simulink model "sampleModel7293_pp_1_1"  (R2018a)
settings: Solver=VariableStepAuto  StartTime=0.0  StopTime=10.0  RelTol=1e-3
undefined symbols (not defined in the file): DiscIntNeverNeededParam
libraries: simulink x367
(part 6 of 12)

== system sampleModel7293_pp_1_1/cfblk167/cfblk17 ==
  cfblk1 : Inport
  Action Port : ActionPort  ActionType=then
  cfblk3 : DiscreteTransferFcn
  cfblk4 : DiscreteIntegrator  SampleTime=-1  OutDataTypeStr=double  ICPrevOutput=DiscIntNeverNeededParam  ICPrevScaledInput=DiscIntNeverNeededParam
  cfblk5 : Subsystem  TreatAsAtomicUnit=on
  cfblk6 : DiscreteZeroPole  Poles=[0 0.5]  Gain=1  SampleTime=-1
  cfblk7 : Subsystem  TreatAsAtomicUnit=on
  cyemi_{112..116} (5 alike) : DataTypeConversion  OutDataTypeStr=double
  emi_417 : Subsystem  TreatAsAtomicUnit=on
  emi_419 : If  IfExpression=Inf <= u1
  emi_420 : DataTypeConversion  OutDataTypeStr=double
  emi_533 : Subsystem  TreatAsAtomicUnit=on
  emi_535 : If  IfExpression=Inf <= u1
  emi_536 : DataTypeConversion  OutDataTypeStr=double
  cfblk2 : Outport
  wires:
  cyemi_112/1 -> cfblk3/1
  cfblk1/1 -> cyemi_112/1
  cyemi_113/1 -> cfblk4/1
  cfblk6/1 -> cyemi_113/1
  cfblk3/1 -> cyemi_114/1, emi_420/1, emi_536/1
  cyemi_115/1 -> cfblk6/1
  cfblk4/1 -> cyemi_116/1
  cyemi_114/1 -> cfblk5/1(emi_415)
  cfblk5/1(emi_416) -> cyemi_115/1
  emi_419/1 -> cfblk5/Action
  emi_419/2 -> emi_417/Action
  emi_420/1 -> emi_419/1
  cyemi_116/1 -> cfblk7/1(emi_531)
  cfblk7/1(emi_532) -> cfblk2/1
  emi_535/1 -> cfblk7/Action
  emi_535/2 -> emi_533/Action
  emi_536/1 -> emi_535/1

== system sampleModel7293_pp_1_1/cfblk167/cfblk18 ==
  cfblk1 : Inport
  cfblk10 : Inport  Port=2
  cfblk11 : Inport  Port=3
  Action Port : ActionPort  ActionType=else
  cfblk14 : Delay
  cfblk3 : simulink/Discrete/Transfer Fcn Lead or Lag  PoleZ=0.95  ZeroZ=0.75  ICPrevOutput=0.0  ICPrevInput=0.0  DoSatur=off
      settings: SourceProductName=Simulink  SourceProductBaseCode=SL
  cfblk4 : Subsystem  TreatAsAtomicUnit=on
  cfblk5 : simulink/Discrete/Tapped Delay  vinit=0.0  samptime=-1  NumDelays=1  DelayOrder=Oldest  includeCurrent=off
  cfblk6 : Subsystem  TreatAsAtomicUnit=on
  cfblk7 : Delay
  cfblk8 : Subsystem  TreatAsAtomicUnit=on
  cfblk9 : DiscreteFir
  cyemi_{120..127} (8 alike) : DataTypeConversion  OutDataTypeStr=double
  emi_1559 : Subsystem  TreatAsAtomicUnit=on
  emi_1561 : If  IfExpression=0 <= u1
  emi_1562 : DataTypeConversion  OutDataTypeStr=double
  emi_2121 : Subsystem  TreatAsAtomicUnit=on
  emi_2123 : If  IfExpression=0 <= u1
  emi_2124 : DataTypeConversion  OutDataTypeStr=double
  emi_38 : Subsystem  TreatAsAtomicUnit=on
  emi_40 : If  IfExpression=0 <= u1
  emi_41 : DataTypeConversion  OutDataTypeStr=double
  cfblk2 : Outport
  cfblk12 : Outport  Port=2
  cfblk13 : Outport  Port=3
  wires:
  cfblk1/1 -> cfblk12/1
  cfblk5/1 -> cfblk2/1, emi_41/1
  cyemi_120/1 -> cfblk14/1
  cfblk9/1 -> cyemi_120/1
  cyemi_121/1 -> cfblk3/1
  cfblk11/1 -> cyemi_121/1
  cyemi_123/1 -> cfblk5/1
  cfblk3/1 -> cyemi_124/1
  cyemi_125/1 -> cfblk7/1
  cfblk14/1 -> cyemi_125/1
  cfblk10/1 -> cyemi_126/1
  cyemi_127/1 -> cfblk9/1
  cfblk7/1 -> cyemi_127/1, emi_2124/1
  cyemi_126/1 -> cfblk8/1(emi_36)
  cfblk8/1(emi_37) -> cfblk13/1, emi_1562/1
  emi_40/1 -> cfblk8/Action
  emi_40/2 -> emi_38/Action
  emi_41/1 -> emi_40/1
  cyemi_122/1 -> cfblk4/1(emi_1557)
  cfblk4/1(emi_1558) -> cyemi_123/1
  emi_1561/1 -> cfblk4/Action
  emi_1561/2 -> emi_1559/Action
  emi_1562/1 -> emi_1561/1
  cyemi_124/1 -> cfblk6/1(emi_2119)
  cfblk6/1(emi_2120) -> cyemi_122/1
  emi_2123/1 -> cfblk6/Action
  emi_2123/2 -> emi_2121/Action
  emi_2124/1 -> emi_2123/1

== system sampleModel7293_pp_1_1/cfblk167/cfblk19 ==
  cfblk1 : Inport
  Action Port : ActionPort  ActionType=then
  cfblk10 : Delay
  cfblk3 : Delay  ShowEnablePort=on
      settings: InputPortMap=u0,e6
  cfblk4 : simulink/Discrete/Transfer Fcn Real Zero  ZeroZ=0.75  ICPrevInput=0.0  DoSatur=off
      settings: SourceProductName=Simulink  SourceProductBaseCode=SL
  cfblk5 : DiscreteZeroPole  Poles=[0 0.5]  Gain=1  SampleTime=-1
  cfblk6 : simulink/Continuous/PID Controller  Controller=PID  TimeDomain=Discrete-time  SampleTime=-1  IntegratorMethod=Forward Euler  FilterMethod=Forward Euler  Form=Parallel  UseFilter=on  ControllerParametersSource=internal  P=1  I=1  D=0  N=100  InitialConditionSource=internal  InitialConditionForIntegrator=0  InitialConditionForFilter=0  ExternalReset=none  LimitOutput=off  UpperSaturationLimit=inf  LowerSaturationLimit=-inf  LinearizeAsGain=off  AntiWindupMode=none  Kb=1  TrackingMode=off  Kt=1  PParamMin=[]  PParamMax=[]  IParamMin=[]  IParamMax=[]  DParamMin=[]  DParamMax=[]  NParamMin=[]  NParamMax=[]  KbParamMin=[]  KbParamMax=[]  KtParamMin=[]  KtParamMax=[]  POutMin=[]  POutMax=[]  IOutMin=[]  IOutMax=[]  DOutMin=[]  DOutMax=[]  NOutMin=[]  NOutMax=[]  KbOutMin=[]  KbOutMax=[]  KtOutMin=[]  KtOutMax=[]  IntegratorOutMin=[]  IntegratorOutMax=[]  FilterOutMin=[]  FilterOutMax=[]  SumOutMin=[]  SumOutMax=[]  SumI1OutMin=[]  SumI1OutMax=[]  SumI2OutMin=[]  SumI2OutMax=[]  SumI3OutMin=[]  SumI3OutMax=[]  SumDOutMin=[]  SumDOutMax=[]  SaturationOutMin=[]  SaturationOutMax=[]  IntegratorContinuousStateAttributes=''  IntegratorStateMustResolveToSignalObject=off  IntegratorRTWStateStorageClass=Auto  FilterContinuousStateAttributes=''  FilterStateMustResolveToSignalObject=off  FilterRTWStateStorageClass=Auto  DifferentiatorICPrevScaledInput=0  DifferentiatorOutMin=[]  DifferentiatorOutMax=[]  FilterDiffOutCoefMin=[]  FilterDiffOutCoefMax=[]  SumDenOutMin=[]  SumDenOutMax=[]  SumNumOutMin=[]  SumNumOutMax=[]  ReciprocalOutMin=[]  ReciprocalOutMax=[]  DivideOutMin=[]  DivideOutMax=[]  TunerSelectOption=Transfer Function Based (PID Tuner App)
  cfblk7 : DiscreteFilter
  cyemi_{129..135} (7 alike) : DataTypeConversion  OutDataTypeStr=double
  cfblk2 : Outport
  cfblk8 : Outport  Port=2
  cfblk9 : Outport  Port=3
  wires:
  cfblk7/1 -> cfblk2/1, cfblk9/1, cyemi_133/1
  cfblk4/1 -> cfblk8/1, cyemi_135/1
  cyemi_129/1 -> cfblk10/1
  cfblk6/1 -> cyemi_129/1
  cyemi_130/1 -> cfblk3/1
  cfblk1/1 -> cyemi_130/1
  cyemi_131/1 -> cfblk3/2
  cfblk10/1 -> cyemi_131/1
  cyemi_132/1 -> cfblk4/1
  cfblk3/1 -> cyemi_132/1
  cyemi_133/1 -> cfblk5/1
  cyemi_134/1 -> cfblk6/1
  cfblk5/1 -> cyemi_134/1
  cyemi_135/1 -> cfblk7/1

== system sampleModel7293_pp_1_1/cfblk167/cfblk20 ==
  cfblk1 : Inport
  cfblk7 : Inport  Port=2
  Action Port : ActionPort  ActionType=else
  cfblk3 : DiscreteStateSpace  SampleTime=-1
  cfblk4 : simulink/Discrete/Transfer Fcn Real Zero  ZeroZ=0.75  ICPrevInput=0.0  DoSatur=off
      settings: SourceProductName=Simulink  SourceProductBaseCode=SL
  cfblk5 : Subsystem  TreatAsAtomicUnit=on
  cfblk6 : Delay  ShowEnablePort=on
      settings: InputPortMap=u0,e6
  cfblk8 : Subsystem  TreatAsAtomicUnit=on
  cyemi_{138..143} (6 alike) : DataTypeConversion  OutDataTypeStr=double
  emi_252 : Subsystem  TreatAsAtomicUnit=on
  emi_254 : If  IfExpression=0 <= u1
  emi_255 : DataTypeConversion  OutDataTypeStr=double
  emi_74 : Subsystem  TreatAsAtomicUnit=on
  emi_76 : If  IfExpression=0 <= u1
  emi_77 : DataTypeConversion  OutDataTypeStr=double
  cfblk2 : Outport
  wires:
  cfblk4/1 -> cfblk2/1
  cyemi_138/1 -> cfblk3/1
  cyemi_139/1 -> cfblk4/1
  cfblk1/1 -> cyemi_140/1
  cyemi_141/1 -> cfblk6/1
  cfblk3/1 -> cyemi_141/1
  cyemi_142/1 -> cfblk6/2
  cfblk7/1 -> cyemi_142/1
  cfblk6/1 -> cyemi_143/1, emi_77/1, emi_255/1
  cyemi_140/1 -> cfblk5/1(emi_72)
  cfblk5/1(emi_73) -> cyemi_139/1
  emi_76/1 -> cfblk5/Action
  emi_76/2 -> emi_74/Action
  emi_77/1 -> emi_76/1
  cyemi_143/1 -> cfblk8/1(emi_250)
  cfblk8/1(emi_251) -> cyemi_138/1
  emi_254/1 -> cfblk8/Action
  emi_254/2 -> emi_252/Action
  emi_255/1 -> emi_254/1

== system sampleModel7293_pp_1_1/cfblk168/cfblk7 ==
  emi_1142 : Inport
  emi_1143 : Inport  Port=2
  Action Port : ActionPort  ActionType=then
  cfblk7 : simulink/Continuous/PID Controller (2DOF)  Controller=PID  TimeDomain=Discrete-time  SampleTime=-1  IntegratorMethod=Forward Euler  FilterMethod=Forward Euler  Form=Parallel  UseFilter=on  ControllerParametersSource=internal  P=1  I=1  D=0  N=100  b=1  c=1  InitialConditionSource=internal  InitialConditionForIntegrator=0  InitialConditionForFilter=0  ExternalReset=none  LimitOutput=off  UpperSaturationLimit=inf  LowerSaturationLimit=-inf  LinearizeAsGain=off  AntiWindupMode=none  Kb=1  TrackingMode=off  Kt=1  PParamMin=[]  PParamMax=[]  IParamMin=[]  IParamMax=[]  DParamMin=[]  DParamMax=[]  NParamMin=[]  NParamMax=[]  bParamMin=[]  bParamMax=[]  cParamMin=[]  cParamMax=[]  KbParamMin=[]  KbParamMax=[]  KtParamMin=[]  KtParamMax=[]  POutMin=[]  POutMax=[]  IOutMin=[]  IOutMax=[]  DOutMin=[]  DOutMax=[]  NOutMin=[]  NOutMax=[]  bOutMin=[]  bOutMax=[]  cOutMin=[]  cOutMax=[]  KbOutMin=[]  KbOutMax=[]  KtOutMin=[]  KtOutMax=[]  IntegratorOutMin=[]  IntegratorOutMax=[]  FilterOutMin=[]  FilterOutMax=[]  SumOutMin=[]  SumOutMax=[]  Sum1OutMin=[]  Sum1OutMax=[]  Sum2OutMin=[]  Sum2OutMax=[]  Sum3OutMin=[]  Sum3OutMax=[]  SumI1OutMin=[]  SumI1OutMax=[]  SumI2OutMin=[]  SumI2OutMax=[]  SumI3OutMin=[]  SumI3OutMax=[]  SumDOutMin=[]  SumDOutMax=[]  SaturationOutMin=[]  SaturationOutMax=[]  IntegratorContinuousStateAttributes=''  IntegratorStateMustResolveToSignalObject=off  IntegratorRTWStateStorageClass=Auto  FilterContinuousStateAttributes=''  FilterStateMustResolveToSignalObject=off  FilterRTWStateStorageClass=Auto  DifferentiatorICPrevScaledInput=0  DifferentiatorOutMin=[]  DifferentiatorOutMax=[]  FilterDiffOutCoefMin=[]  FilterDiffOutCoefMax=[]  SumDenOutMin=[]  SumDenOutMax=[]  SumNumOutMin=[]  SumNumOutMax=[]  ReciprocalOutMin=[]  ReciprocalOutMax=[]  DivideOutMin=[]  DivideOutMax=[]  TunerSelectOption=Transfer Function Based (PID Tuner App)
  emi_1144 : Outport
  wires:
  emi_1142/1 -> cfblk7/1
  emi_1143/1 -> cfblk7/2
  cfblk7/1 -> emi_1144/1

== system sampleModel7293_pp_1_1/cfblk168/emi_1145 ==
  Action Port : ActionPort  ActionType=else
  emi_1146 : Assertion

== system sampleModel7293_pp_1_1/cfblk169/cfblk3 ==
  emi_1128 : Inport
  Action Port : ActionPort  ActionType=then
  cfblk3 : DiscreteFilter
  emi_1129 : Outport
  wires:
  emi_1128/1 -> cfblk3/1
  cfblk3/1 -> emi_1129/1

== system sampleModel7293_pp_1_1/cfblk169/cfblk5 ==
  emi_825 : Inport
  Action Port : ActionPort  ActionType=then
  cfblk5 : DiscreteFir
  emi_826 : Outport
  wires:
  emi_825/1 -> cfblk5/1
  cfblk5/1 -> emi_826/1

== system sampleModel7293_pp_1_1/cfblk169/cfblk7 ==
  emi_1976 : Inport
  Action Port : ActionPort  ActionType=then
  cfblk7 : DiscreteStateSpace  SampleTime=-1
  emi_1977 : Outport
  wires:
  emi_1976/1 -> cfblk7/1
  cfblk7/1 -> emi_1977/1

== system sampleModel7293_pp_1_1/cfblk169/cfblk8 ==
  emi_487 : Inport
  emi_488 : Inport  Port=2
  Action Port : ActionPort  ActionType=then
  cfblk8 : Delay  ShowEnablePort=on
      settings: InputPortMap=u0,e6
  emi_489 : Outport
  wires:
  emi_487/1 -> cfblk8/1
  emi_488/1 -> cfblk8/2
  cfblk8/1 -> emi_489/1

== system sampleModel7293_pp_1_1/cfblk169/cfblk9 ==
  emi_294 : Inport
  Action Port : ActionPort  ActionType=then
  cfblk9 : DiscreteIntegrator  SampleTime=-1  OutDataTypeStr=double  ICPrevOutput=DiscIntNeverNeededParam  ICPrevScaledInput=DiscIntNeverNeededParam
  emi_295 : Outport
  wires:
  emi_294/1 -> cfblk9/1
  cfblk9/1 -> emi_295/1

== system sampleModel7293_pp_1_1/cfblk169/emi_1130 ==
  Action Port : ActionPort  ActionType=else
  emi_1131 : Assertion

== system sampleModel7293_pp_1_1/cfblk169/emi_1978 ==
  Action Port : ActionPort  ActionType=else
  emi_1979 : Assertion

== system sampleModel7293_pp_1_1/cfblk169/emi_296 ==
  Action Port : ActionPort  ActionType=else
  emi_297 : Assertion

== system sampleModel7293_pp_1_1/cfblk169/emi_490 ==
  Action Port : ActionPort  ActionType=else
  emi_491 : Assertion

== system sampleModel7293_pp_1_1/cfblk169/emi_827 ==
  Action Port : ActionPort  ActionType=else
  emi_828 : Assertion

== system sampleModel7293_pp_1_1/cfblk170/cfblk14 ==
  cfblk1 : Inport
  Action Port : ActionPort  ActionType=then
  cfblk3 : DiscreteTransferFcn
  cfblk4 : DiscreteTransferFcn
  cfblk5 : Subsystem  TreatAsAtomicUnit=on
  cfblk6 : DiscreteStateSpace  SampleTime=-1
  cfblk8 : Subsystem  TreatAsAtomicUnit=on
  cyemi_{187..192} (6 alike) : DataTypeConversion  OutDataTypeStr=double
  emi_1667 : Subsystem  TreatAsAtomicUnit=on
  emi_1669 : If  IfExpression=Inf <= u1
  emi_1670 : DataTypeConversion  OutDataTypeStr=double
  emi_669 : Subsystem  TreatAsAtomicUnit=on
  emi_671 : If  IfExpression=Inf <= u1
  emi_672 : DataTypeConversion  OutDataTypeStr=double
  cfblk2 : Outport
  cfblk7 : Outport  Port=2
  wires:
  cfblk3/1 -> cfblk2/1
  cfblk1/1 -> cfblk7/1
  cyemi_187/1 -> cfblk3/1
  cfblk6/1 -> cyemi_187/1, emi_672/1
  cyemi_188/1 -> cfblk4/1
  cfblk4/1 -> cyemi_189/1, cyemi_190/1
  cyemi_191/1 -> cfblk6/1
  cyemi_192/1 -> cfblk8/1(emi_667)
  cfblk8/1(emi_668) -> cyemi_188/1, emi_1670/1
  emi_671/1 -> cfblk8/Action
  emi_671/2 -> emi_669/Action
  emi_672/1 -> emi_671/1
  cyemi_189/1 -> cfblk5/1(emi_1664)
  cyemi_190/1 -> cfblk5/2(emi_1665)
  cfblk5/1(emi_1666) -> cyemi_192/1, cyemi_191/1
  emi_1669/1 -> cfblk5/Action
  emi_1669/2 -> emi_1667/Action
  emi_1670/1 -> emi_1669/1

== system sampleModel7293_pp_1_1/cfblk170/cfblk15 ==
  cfblk1 : Inport
  cfblk8 : Inport  Port=2
  Action Port : ActionPort  ActionType=else
  cfblk10 : Delay
  cfblk3 : DiscreteIntegrator  SampleTime=-1  OutDataTypeStr=double  ICPrevOutput=DiscIntNeverNeededParam  ICPrevScaledInput=DiscIntNeverNeededParam
  cfblk4 : Subsystem  TreatAsAtomicUnit=on
  cfblk5 : Subsystem  TreatAsAtomicUnit=on
  cfblk6 : DiscreteFilter
  cfblk7 : Subsystem  TreatAsAtomicUnit=on
  cfblk9 : Delay
  cyemi_{195..202} (8 alike) : DataTypeConversion  OutDataTypeStr=double
  emi_1845 : Subsystem  TreatAsAtomicUnit=on
  emi_1847 : If  IfExpression=0 <= u1
  emi_1848 : DataTypeConversion  OutDataTypeStr=double
  emi_1866 : Subsystem  TreatAsAtomicUnit=on
  emi_1868 : If  IfExpression=0 <= u1
  emi_1869 : DataTypeConversion  OutDataTypeStr=double
  emi_188 : Subsystem  TreatAsAtomicUnit=on
  emi_190 : If  IfExpression=0 <= u1
  emi_191 : DataTypeConversion  OutDataTypeStr=double
  cfblk2 : Outport
  wires:
  cfblk1/1 -> cfblk2/1
  cyemi_195/1 -> cfblk10/1
  cfblk6/1 -> cyemi_195/1
  cyemi_196/1 -> cfblk3/1
  cfblk9/1 -> cyemi_196/1, emi_1848/1, emi_1869/1
  cfblk10/1 -> cyemi_197/1, emi_191/1
  cfblk3/1 -> cyemi_198/1
  cyemi_199/1 -> cfblk6/1
  cfblk8/1 -> cyemi_201/1
  cyemi_202/1 -> cfblk9/1
  cyemi_200/1 -> cfblk7/1(emi_185)
  cyemi_201/1 -> cfblk7/2(emi_186)
  cfblk7/1(emi_187) -> cyemi_202/1
  emi_190/1 -> cfblk7/Action
  emi_190/2 -> emi_188/Action
  emi_191/1 -> emi_190/1
  cyemi_198/1 -> cfblk5/1(emi_1843)
  cfblk5/1(emi_1844) -> cyemi_200/1
  emi_1847/1 -> cfblk5/Action
  emi_1847/2 -> emi_1845/Action
  emi_1848/1 -> emi_1847/1
  cyemi_197/1 -> cfblk4/1(emi_1864)
  cfblk4/1(emi_1865) -> cyemi_199/1
  emi_1868/1 -> cfblk4/Action
  emi_1868/2 -> emi_1866/Action
  emi_1869/1 -> emi_1868/1

== system sampleModel7293_pp_1_1/cfblk170/cfblk16 ==
  cfblk1 : Inport
  Action Port : ActionPort  ActionType=then
  cfblk10 : DiscreteZeroPole  Poles=[0 0.5]  Gain=1  SampleTime=-1
  cfblk11 : DiscreteFir
  cfblk12 : Delay
  cfblk3 : Subsystem  TreatAsAtomicUnit=on
  cfblk4 : simulink/Continuous/PID Controller  Controller=PID  TimeDomain=Discrete-time  SampleTime=-1  IntegratorMethod=Forward Euler  FilterMethod=Forward Euler  Form=Parallel  UseFilter=on  ControllerParametersSource=internal  P=1  I=1  D=0  N=100  InitialConditionSource=internal  InitialConditionForIntegrator=0  InitialConditionForFilter=0  ExternalReset=none  LimitOutput=off  UpperSaturationLimit=inf  LowerSaturationLimit=-inf  LinearizeAsGain=off  AntiWindupMode=none  Kb=1  TrackingMode=off  Kt=1  PParamMin=[]  PParamMax=[]  IParamMin=[]  IParamMax=[]  DParamMin=[]  DParamMax=[]  NParamMin=[]  NParamMax=[]  KbParamMin=[]  KbParamMax=[]  KtParamMin=[]  KtParamMax=[]  POutMin=[]  POutMax=[]  IOutMin=[]  IOutMax=[]  DOutMin=[]  DOutMax=[]  NOutMin=[]  NOutMax=[]  KbOutMin=[]  KbOutMax=[]  KtOutMin=[]  KtOutMax=[]  IntegratorOutMin=[]  IntegratorOutMax=[]  FilterOutMin=[]  FilterOutMax=[]  SumOutMin=[]  SumOutMax=[]  SumI1OutMin=[]  SumI1OutMax=[]  SumI2OutMin=[]  SumI2OutMax=[]  SumI3OutMin=[]  SumI3OutMax=[]  SumDOutMin=[]  SumDOutMax=[]  SaturationOutMin=[]  SaturationOutMax=[]  IntegratorContinuousStateAttributes=''  IntegratorStateMustResolveToSignalObject=off  IntegratorRTWStateStorageClass=Auto  FilterContinuousStateAttributes=''  FilterStateMustResolveToSignalObject=off  FilterRTWStateStorageClass=Auto  DifferentiatorICPrevScaledInput=0  DifferentiatorOutMin=[]  DifferentiatorOutMax=[]  FilterDiffOutCoefMin=[]  FilterDiffOutCoefMax=[]  SumDenOutMin=[]  SumDenOutMax=[]  SumNumOutMin=[]  SumNumOutMax=[]  ReciprocalOutMin=[]  ReciprocalOutMax=[]  DivideOutMin=[]  DivideOutMax=[]  TunerSelectOption=Transfer Function Based (PID Tuner App)
  cfblk5 : simulink/Continuous/PID Controller  Controller=PID  TimeDomain=Discrete-time  SampleTime=-1  IntegratorMethod=Forward Euler  FilterMethod=Forward Euler  Form=Parallel  UseFilter=on  ControllerParametersSource=internal  P=1  I=1  D=0  N=100  InitialConditionSource=internal  InitialConditionForIntegrator=0  InitialConditionForFilter=0  ExternalReset=none  LimitOutput=off  UpperSaturationLimit=inf  LowerSaturationLimit=-inf  LinearizeAsGain=off  AntiWindupMode=none  Kb=1  TrackingMode=off  Kt=1  PParamMin=[]  PParamMax=[]  IParamMin=[]  IParamMax=[]  DParamMin=[]  DParamMax=[]  NParamMin=[]  NParamMax=[]  KbParamMin=[]  KbParamMax=[]  KtParamMin=[]  KtParamMax=[]  POutMin=[]  POutMax=[]  IOutMin=[]  IOutMax=[]  DOutMin=[]  DOutMax=[]  NOutMin=[]  NOutMax=[]  KbOutMin=[]  KbOutMax=[]  KtOutMin=[]  KtOutMax=[]  IntegratorOutMin=[]  IntegratorOutMax=[]  FilterOutMin=[]  FilterOutMax=[]  SumOutMin=[]  SumOutMax=[]  SumI1OutMin=[]  SumI1OutMax=[]  SumI2OutMin=[]  SumI2OutMax=[]  SumI3OutMin=[]  SumI3OutMax=[]  SumDOutMin=[]  SumDOutMax=[]  SaturationOutMin=[]  SaturationOutMax=[]  IntegratorContinuousStateAttributes=''  IntegratorStateMustResolveToSignalObject=off  IntegratorRTWStateStorageClass=Auto  FilterContinuousStateAttributes=''  FilterStateMustResolveToSignalObject=off  FilterRTWStateStorageClass=Auto  DifferentiatorICPrevScaledInput=0  DifferentiatorOutMin=[]  DifferentiatorOutMax=[]  FilterDiffOutCoefMin=[]  FilterDiffOutCoefMax=[]  SumDenOutMin=[]  SumDenOutMax=[]  SumNumOutMin=[]  SumNumOutMax=[]  ReciprocalOutMin=[]  ReciprocalOutMax=[]  DivideOutMin=[]  DivideOutMax=[]  TunerSelectOption=Transfer Function Based (PID Tuner App)
  cfblk6 : DiscreteFilter
  cfblk7 : DiscreteTransferFcn
  cfblk8 : simulink/Continuous/PID Controller (2DOF)  Controller=PID  TimeDomain=Discrete-time  SampleTime=-1  IntegratorMethod=Forward Euler  FilterMethod=Forward Euler  Form=Parallel  UseFilter=on  ControllerParametersSource=internal  P=1  I=1  D=0  N=100  b=1  c=1  InitialConditionSource=internal  InitialConditionForIntegrator=0  InitialConditionForFilter=0  ExternalReset=none  LimitOutput=off  UpperSaturationLimit=inf  LowerSaturationLimit=-inf  LinearizeAsGain=off  AntiWindupMode=none  Kb=1  TrackingMode=off  Kt=1  PParamMin=[]  PParamMax=[]  IParamMin=[]  IParamMax=[]  DParamMin=[]  DParamMax=[]  NParamMin=[]  NParamMax=[]  bParamMin=[]  bParamMax=[]  cParamMin=[]  cParamMax=[]  KbParamMin=[]  KbParamMax=[]  KtParamMin=[]  KtParamMax=[]  POutMin=[]  POutMax=[]  IOutMin=[]  IOutMax=[]  DOutMin=[]  DOutMax=[]  NOutMin=[]  NOutMax=[]  bOutMin=[]  bOutMax=[]  cOutMin=[]  cOutMax=[]  KbOutMin=[]  KbOutMax=[]  KtOutMin=[]  KtOutMax=[]  IntegratorOutMin=[]  IntegratorOutMax=[]  FilterOutMin=[]  FilterOutMax=[]  SumOutMin=[]  SumOutMax=[]  Sum1OutMin=[]  Sum1OutMax=[]  Sum2OutMin=[]  Sum2OutMax=[]  Sum3OutMin=[]  Sum3OutMax=[]  SumI1OutMin=[]  SumI1OutMax=[]  SumI2OutMin=[]  SumI2OutMax=[]  SumI3OutMin=[]  SumI3OutMax=[]  SumDOutMin=[]  SumDOutMax=[]  SaturationOutMin=[]  SaturationOutMax=[]  IntegratorContinuousStateAttributes=''  IntegratorStateMustResolveToSignalObject=off  IntegratorRTWStateStorageClass=Auto  FilterContinuousStateAttributes=''  FilterStateMustResolveToSignalObject=off  FilterRTWStateStorageClass=Auto  DifferentiatorICPrevScaledInput=0  DifferentiatorOutMin=[]  DifferentiatorOutMax=[]  FilterDiffOutCoefMin=[]  FilterDiffOutCoefMax=[]  SumDenOutMin=[]  SumDenOutMax=[]  SumNumOutMin=[]  SumNumOutMax=[]  ReciprocalOutMin=[]  ReciprocalOutMax=[]  DivideOutMin=[]  DivideOutMax=[]  TunerSelectOption=Transfer Function Based (PID Tuner App)
  cfblk9 : UnitDelay  SampleTime=-1
  cyemi_{204..214} (11 alike) : DataTypeConversion  OutDataTypeStr=double
  emi_1638 : Subsystem  TreatAsAtomicUnit=on
  emi_1640 : If  IfExpression=Inf <= u1
  emi_1641 : DataTypeConversion  OutDataTypeStr=double
  cfblk2 : Outport
  wires:
  cyemi_204/1 -> cfblk10/1
  cfblk1/1 -> cyemi_204/1
  cyemi_205/1 -> cfblk11/1
  cfblk8/1 -> cyemi_205/1
  cyemi_206/1 -> cfblk12/1
  cfblk4/1 -> cyemi_206/1
  cfblk10/1 -> cyemi_207/1
  cyemi_208/1 -> cfblk4/1
  cfblk9/1 -> cyemi_208/1
  cyemi_209/1 -> cfblk5/1
  cfblk7/1 -> cyemi_209/1
  cyemi_210/1 -> cfblk6/1
  cfblk5/1 -> cyemi_210/1
  cyemi_211/1 -> cfblk7/1
  cyemi_212/1 -> cfblk8/1
  cfblk6/1 -> cyemi_212/1, emi_1641/1
  cyemi_213/1 -> cfblk8/2
  cfblk12/1 -> cyemi_213/1
  cyemi_214/1 -> cfblk9/1
  cfblk11/1 -> cyemi_214/1
  cyemi_207/1 -> cfblk3/1(emi_1636)
  cfblk3/1(emi_1637) -> cyemi_211/1, cfblk2/1
  emi_1640/1 -> cfblk3/Action
  emi_1640/2 -> emi_1638/Action
  emi_1641/1 -> emi_1640/1

== system sampleModel7293_pp_1_1/cfblk170/cfblk17 ==
  cfblk1 : Inport
  cfblk10 : Inport  Port=2
  cfblk11 : Inport  Port=3
  cfblk12 : Inport  Port=4
  cfblk13 : Inport  Port=5
  Action Port : ActionPort  ActionType=else
  cfblk3 : Subsystem  TreatAsAtomicUnit=on
  cfblk4 : simulink/Discrete/Transfer Fcn Lead or Lag  PoleZ=0.95  ZeroZ=0.75  ICPrevOutput=0.0  ICPrevInput=0.0  DoSatur=off
      settings: SourceProductName=Simulink  SourceProductBaseCode=SL
  cfblk5 : DiscreteIntegrator  SampleTime=-1  OutDataTypeStr=double  ICPrevOutput=DiscIntNeverNeededParam  ICPrevScaledInput=DiscIntNeverNeededParam
  cfblk6 : simulink/Continuous/PID Controller (2DOF)  Controller=PID  TimeDomain=Discrete-time  SampleTime=-1  IntegratorMethod=Forward Euler  FilterMethod=Forward Euler  Form=Parallel  UseFilter=on  ControllerParametersSource=internal  P=1  I=1  D=0  N=100  b=1  c=1  InitialConditionSource=internal  InitialConditionForIntegrator=0  InitialConditionForFilter=0  ExternalReset=none  LimitOutput=off  UpperSaturationLimit=inf  LowerSaturationLimit=-inf  LinearizeAsGain=off  AntiWindupMode=none  Kb=1  TrackingMode=off  Kt=1  PParamMin=[]  PParamMax=[]  IParamMin=[]  IParamMax=[]  DParamMin=[]  DParamMax=[]  NParamMin=[]  NParamMax=[]  bParamMin=[]  bParamMax=[]  cParamMin=[]  cParamMax=[]  KbParamMin=[]  KbParamMax=[]  KtParamMin=[]  KtParamMax=[]  POutMin=[]  POutMax=[]  IOutMin=[]  IOutMax=[]  DOutMin=[]  DOutMax=[]  NOutMin=[]  NOutMax=[]  bOutMin=[]  bOutMax=[]  cOutMin=[]  cOutMax=[]  KbOutMin=[]  KbOutMax=[]  KtOutMin=[]  KtOutMax=[]  IntegratorOutMin=[]  IntegratorOutMax=[]  FilterOutMin=[]  FilterOutMax=[]  SumOutMin=[]  SumOutMax=[]  Sum1OutMin=[]  Sum1OutMax=[]  Sum2OutMin=[]  Sum2OutMax=[]  Sum3OutMin=[]  Sum3OutMax=[]  SumI1OutMin=[]  SumI1OutMax=[]  SumI2OutMin=[]  SumI2OutMax=[]  SumI3OutMin=[]  SumI3OutMax=[]  SumDOutMin=[]  SumDOutMax=[]  SaturationOutMin=[]  SaturationOutMax=[]  IntegratorContinuousStateAttributes=''  IntegratorStateMustResolveToSignalObject=off  IntegratorRTWStateStorageClass=Auto  FilterContinuousStateAttributes=''  FilterStateMustResolveToSignalObject=off  FilterRTWStateStorageClass=Auto  DifferentiatorICPrevScaledInput=0  DifferentiatorOutMin=[]  DifferentiatorOutMax=[]  FilterDiffOutCoefMin=[]  FilterDiffOutCoefMax=[]  SumDenOutMin=[]  SumDenOutMax=[]  SumNumOutMin=[]  SumNumOutMax=[]  ReciprocalOutMin=[]  ReciprocalOutMax=[]  DivideOutMin=[]  DivideOutMax=[]  TunerSelectOption=Transfer Function Based (PID Tuner App)
  cfblk7 : simulink/Discrete/Tapped Delay  vinit=0.0  samptime=-1  NumDelays=1  DelayOrder=Oldest  includeCurrent=off
  cfblk8 : Delay
  cfblk9 : DiscreteStateSpace  SampleTime=-1
  cyemi_{220..227} (8 alike) : DataTypeConversion  OutDataTypeStr=double
  emi_1631 : Subsystem  TreatAsAtomicUnit=on
  emi_1633 : If  IfExpression=0 <= u1
  emi_1634 : DataTypeConversion  OutDataTypeStr=double
  cfblk2 : Outport
  wires:
  cfblk6/1 -> cfblk2/1
  cfblk4/1 -> cyemi_220/1
  cyemi_221/1 -> cfblk4/1
  cfblk9/1 -> cyemi_221/1, emi_1634/1
  cyemi_222/1 -> cfblk5/1
  cyemi_223/1 -> cfblk6/1
  cfblk11/1 -> cyemi_223/1
  cyemi_224/1 -> cfblk6/2
  cfblk5/1 -> cyemi_224/1
  cyemi_225/1 -> cfblk7/1
  cfblk12/1 -> cyemi_225/1
  cyemi_226/1 -> cfblk8/1
  cfblk10/1 -> cyemi_226/1
  cyemi_227/1 -> cfblk9/1
  cfblk7/1 -> cyemi_227/1
  cyemi_220/1 -> cfblk3/1(emi_1629)
  cfblk3/1(emi_1630) -> cyemi_222/1
  emi_1633/1 -> cfblk3/Action
  emi_1633/2 -> emi_1631/Action
  emi_1634/1 -> emi_1633/1

== system sampleModel7293_pp_1_1/cfblk170/cfblk21 ==
  emi_1415 : Inport
  Action Port : ActionPort  ActionType=then
  cfblk21 : Delay
  emi_1416 : Outport
  wires:
  emi_1415/1 -> cfblk21/1
  cfblk21/1 -> emi_1416/1

== system sampleModel7293_pp_1_1/cfblk170/cfblk3 ==
  emi_2068 : Inport
  Action Port : ActionPort  ActionType=then
  cfblk3 : DiscreteStateSpace  SampleTime=-1
  emi_2069 : Outport
  wires:
  emi_2068/1 -> cfblk3/1
  cfblk3/1 -> emi_2069/1

== system sampleModel7293_pp_1_1/cfblk170/cfblk4 ==
  emi_86 : Inport
  emi_87 : Inport  Port=2
  Action Port : ActionPort  ActionType=then
  cfblk4 : simulink/Continuous/PID Controller (2DOF)  Controller=PID  TimeDomain=Discrete-time  SampleTime=-1  IntegratorMethod=Forward Euler  FilterMethod=Forward Euler  Form=Parallel  UseFilter=on  ControllerParametersSource=internal  P=1  I=1  D=0  N=100  b=1  c=1  InitialConditionSource=internal  InitialConditionForIntegrator=0  InitialConditionForFilter=0  ExternalReset=none  LimitOutput=off  UpperSaturationLimit=inf  LowerSaturationLimit=-inf  LinearizeAsGain=off  AntiWindupMode=none  Kb=1  TrackingMode=off  Kt=1  PParamMin=[]  PParamMax=[]  IParamMin=[]  IParamMax=[]  DParamMin=[]  DParamMax=[]  NParamMin=[]  NParamMax=[]  bParamMin=[]  bParamMax=[]  cParamMin=[]  cParamMax=[]  KbParamMin=[]  KbParamMax=[]  KtParamMin=[]  KtParamMax=[]  POutMin=[]  POutMax=[]  IOutMin=[]  IOutMax=[]  DOutMin=[]  DOutMax=[]  NOutMin=[]  NOutMax=[]  bOutMin=[]  bOutMax=[]  cOutMin=[]  cOutMax=[]  KbOutMin=[]  KbOutMax=[]  KtOutMin=[]  KtOutMax=[]  IntegratorOutMin=[]  IntegratorOutMax=[]  FilterOutMin=[]  FilterOutMax=[]  SumOutMin=[]  SumOutMax=[]  Sum1OutMin=[]  Sum1OutMax=[]  Sum2OutMin=[]  Sum2OutMax=[]  Sum3OutMin=[]  Sum3OutMax=[]  SumI1OutMin=[]  SumI1OutMax=[]  SumI2OutMin=[]  SumI2OutMax=[]  SumI3OutMin=[]  SumI3OutMax=[]  SumDOutMin=[]  SumDOutMax=[]  SaturationOutMin=[]  SaturationOutMax=[]  IntegratorContinuousStateAttributes=''  IntegratorStateMustResolveToSignalObject=off  IntegratorRTWStateStorageClass=Auto  FilterContinuousStateAttributes=''  FilterStateMustResolveToSignalObject=off  FilterRTWStateStorageClass=Auto  DifferentiatorICPrevScaledInput=0  DifferentiatorOutMin=[]  DifferentiatorOutMax=[]  FilterDiffOutCoefMin=[]  FilterDiffOutCoefMax=[]  SumDenOutMin=[]  SumDenOutMax=[]  SumNumOutMin=[]  SumNumOutMax=[]  ReciprocalOutMin=[]  ReciprocalOutMax=[]  DivideOutMin=[]  DivideOutMax=[]  TunerSelectOption=Transfer Function Based (PID Tuner App)
  emi_88 : Outport
  wires:
  emi_86/1 -> cfblk4/1
  emi_87/1 -> cfblk4/2
  cfblk4/1 -> emi_88/1

== system sampleModel7293_pp_1_1/cfblk170/cfblk5 ==
  emi_344 : Inport
  emi_345 : Inport  Port=2
  Action Port : ActionPort  ActionType=then
  cfblk5 : Delay  ShowEnablePort=on
      settings: InputPortMap=u0,e6
  emi_346 : Outport
  wires:
  emi_344/1 -> cfblk5/1
  emi_345/1 -> cfblk5/2
  cfblk5/1 -> emi_346/1

== system sampleModel7293_pp_1_1/cfblk170/cfblk7 ==
  emi_1280 : Inport
  Action Port : ActionPort  ActionType=then
  cfblk7 : Delay
  emi_1281 : Outport
  wires:
  emi_1280/1 -> cfblk7/1
  cfblk7/1 -> emi_1281/1

== system sampleModel7293_pp_1_1/cfblk170/cfblk8 ==
  emi_1121 : Inport
  Action Port : ActionPort  ActionType=then
  cfblk8 : DiscreteFilter
  emi_1122 : Outport
  wires:
  emi_1121/1 -> cfblk8/1
  cfblk8/1 -> emi_1122/1

== system sampleModel7293_pp_1_1/cfblk170/emi_1123 ==
  Action Port : ActionPort  ActionType=else
  emi_1124 : Assertion

== system sampleModel7293_pp_1_1/cfblk170/emi_1282 ==
  Action Port : ActionPort  ActionType=else
  emi_1283 : Assertion

== system sampleModel7293_pp_1_1/cfblk170/emi_1417 ==
  Action Port : ActionPort  ActionType=else
  emi_1418 : Assertion

== system sampleModel7293_pp_1_1/cfblk170/emi_2070 ==
  Action Port : ActionPort  ActionType=else
  emi_2071 : Assertion

== system sampleModel7293_pp_1_1/cfblk170/emi_347 ==
  Action Port : ActionPort  ActionType=else
  emi_348 : Assertion

== system sampleModel7293_pp_1_1/cfblk170/emi_89 ==
  Action Port : ActionPort  ActionType=else
  emi_90 : Assertion

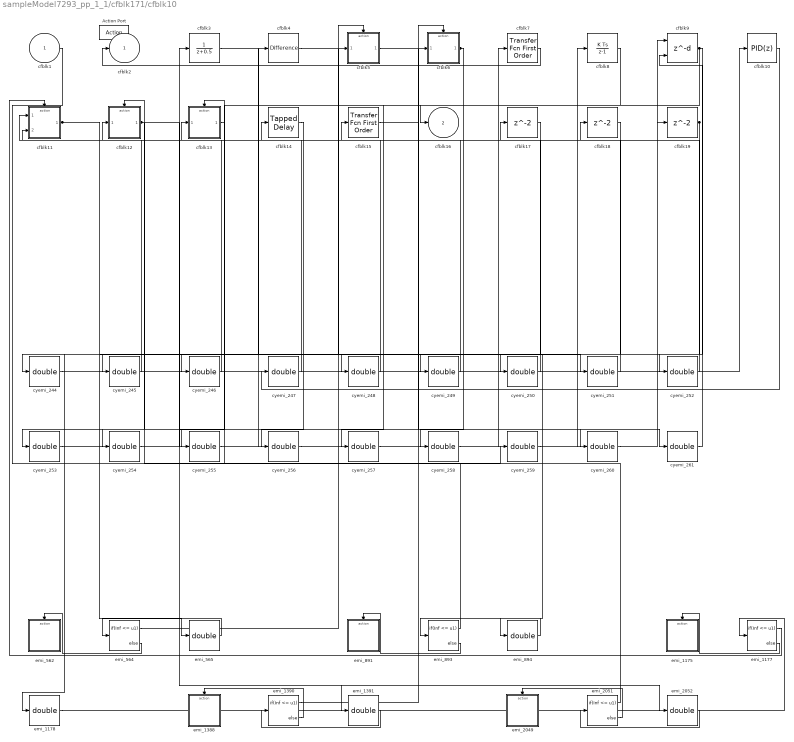
== system sampleModel7293_pp_1_1/cfblk171/cfblk10 ==
  cfblk1 : Inport
  Action Port : ActionPort  ActionType=then
  cfblk10 : simulink/Continuous/PID Controller  Controller=PID  TimeDomain=Discrete-time  SampleTime=-1  IntegratorMethod=Forward Euler  FilterMethod=Forward Euler  Form=Parallel  UseFilter=on  ControllerParametersSource=internal  P=1  I=1  D=0  N=100  InitialConditionSource=internal  InitialConditionForIntegrator=0  InitialConditionForFilter=0  ExternalReset=none  LimitOutput=off  UpperSaturationLimit=inf  LowerSaturationLimit=-inf  LinearizeAsGain=off  AntiWindupMode=none  Kb=1  TrackingMode=off  Kt=1  PParamMin=[]  PParamMax=[]  IParamMin=[]  IParamMax=[]  DParamMin=[]  DParamMax=[]  NParamMin=[]  NParamMax=[]  KbParamMin=[]  KbParamMax=[]  KtParamMin=[]  KtParamMax=[]  POutMin=[]  POutMax=[]  IOutMin=[]  IOutMax=[]  DOutMin=[]  DOutMax=[]  NOutMin=[]  NOutMax=[]  KbOutMin=[]  KbOutMax=[]  KtOutMin=[]  KtOutMax=[]  IntegratorOutMin=[]  IntegratorOutMax=[]  FilterOutMin=[]  FilterOutMax=[]  SumOutMin=[]  SumOutMax=[]  SumI1OutMin=[]  SumI1OutMax=[]  SumI2OutMin=[]  SumI2OutMax=[]  SumI3OutMin=[]  SumI3OutMax=[]  SumDOutMin=[]  SumDOutMax=[]  SaturationOutMin=[]  SaturationOutMax=[]  IntegratorContinuousStateAttributes=''  IntegratorStateMustResolveToSignalObject=off  IntegratorRTWStateStorageClass=Auto  FilterContinuousStateAttributes=''  FilterStateMustResolveToSignalObject=off  FilterRTWStateStorageClass=Auto  DifferentiatorICPrevScaledInput=0  DifferentiatorOutMin=[]  DifferentiatorOutMax=[]  FilterDiffOutCoefMin=[]  FilterDiffOutCoefMax=[]  SumDenOutMin=[]  SumDenOutMax=[]  SumNumOutMin=[]  SumNumOutMax=[]  ReciprocalOutMin=[]  ReciprocalOutMax=[]  DivideOutMin=[]  DivideOutMax=[]  TunerSelectOption=Transfer Function Based (PID Tuner App)
  cfblk11 : Subsystem  TreatAsAtomicUnit=on
  cfblk12 : Subsystem  TreatAsAtomicUnit=on
  cfblk13 : Subsystem  TreatAsAtomicUnit=on
  cfblk14 : simulink/Discrete/Tapped Delay  vinit=0.0  samptime=-1  NumDelays=1  DelayOrder=Oldest  includeCurrent=off
  cfblk15 : simulink/Discrete/Transfer Fcn First Order  PoleZ=0.95  ICPrevOutput=0.0  DoSatur=off
      settings: SourceProductName=Simulink
  cfblk17 : Delay
  cfblk18 : Delay
  cfblk19 : Delay
  cfblk3 : DiscreteTransferFcn
  cfblk4 : simulink/Discrete/Difference  ICPrevInput=0.0  OutMin=[]  OutMax=[]  OutDataTypeStr=double  OutputDataTypeScalingMode=double  OutDataType=fixdt(1, 16)  OutScaling=2^-10  DoSatur=off
  cfblk5 : Subsystem  TreatAsAtomicUnit=on
  cfblk6 : Subsystem  TreatAsAtomicUnit=on
  cfblk7 : simulink/Discrete/Transfer Fcn First Order  PoleZ=0.95  ICPrevOutput=0.0  DoSatur=off
      settings: SourceProductName=Simulink
  cfblk8 : DiscreteIntegrator  SampleTime=-1  OutDataTypeStr=double  ICPrevOutput=DiscIntNeverNeededParam  ICPrevScaledInput=DiscIntNeverNeededParam
  cfblk9 : Delay  DelayLengthSource=Input port
      settings: InputPortMap=u0,p1
  cyemi_{244..261} (18 alike) : DataTypeConversion  OutDataTypeStr=double
  emi_1175 : Subsystem  TreatAsAtomicUnit=on
  emi_{564,893,1177,1390,2051} (5 alike) : If  IfExpression=Inf <= u1
  emi_{565,894,1178,1391,2052} (5 alike) : DataTypeConversion  OutDataTypeStr=double
  emi_1388 : Subsystem  TreatAsAtomicUnit=on
  emi_2049 : Subsystem  TreatAsAtomicUnit=on
  emi_562 : Subsystem  TreatAsAtomicUnit=on
  emi_891 : Subsystem  TreatAsAtomicUnit=on
  cfblk2 : Outport
  cfblk16 : Outport  Port=2
  wires:
  cfblk7/1 -> cfblk2/1
  cfblk9/1 -> cyemi_252/1, cyemi_257/1
  cyemi_244/1 -> cfblk10/1
  cfblk19/1 -> cyemi_244/1, emi_894/1, emi_1178/1
  cfblk17/1 -> cyemi_245/1
  cfblk8/1 -> cyemi_246/1
  cfblk10/1 -> cyemi_247/1
  cyemi_249/1 -> cfblk14/1
  cfblk4/1 -> cyemi_249/1
  cyemi_250/1 -> cfblk15/1
  cyemi_251/1 -> cfblk17/1
  cfblk3/1 -> cyemi_251/1
  cyemi_252/1 -> cfblk18/1
  cyemi_253/1 -> cfblk19/1
  cyemi_254/1 -> cfblk3/1
  cyemi_255/1 -> cfblk4/1
  cfblk18/1 -> cyemi_255/1
  cfblk14/1 -> cyemi_256/1
  cyemi_258/1 -> cfblk7/1
  cyemi_259/1 -> cfblk8/1
  cfblk1/1 -> cyemi_259/1
  cyemi_260/1 -> cfblk9/1
  cfblk15/1 -> cyemi_260/1
  cyemi_261/1 -> cfblk9/2
  cyemi_256/1 -> cfblk5/1(emi_560)
  cfblk5/1(emi_561) -> cyemi_250/1
  emi_564/1 -> cfblk5/Action
  emi_564/2 -> emi_562/Action
  emi_565/1 -> emi_564/1
  cyemi_247/1 -> cfblk12/1(emi_889)
  cfblk12/1(emi_890) -> cyemi_261/1, cyemi_253/1, emi_1391/1, emi_2052/1
  emi_893/1 -> cfblk12/Action
  emi_893/2 -> emi_891/Action
  emi_894/1 -> emi_893/1
  cyemi_245/1 -> cfblk11/1(emi_1172)
  cyemi_246/1 -> cfblk11/2(emi_1173)
  cfblk11/1(emi_1174) -> emi_565/1, cyemi_248/1
  emi_1177/1 -> cfblk11/Action
  emi_1177/2 -> emi_1175/Action
  emi_1178/1 -> emi_1177/1
  cyemi_257/1 -> cfblk6/1(emi_1386)
  cfblk6/1(emi_1387) -> cyemi_258/1, cfblk16/1
  emi_1390/1 -> cfblk6/Action
  emi_1390/2 -> emi_1388/Action
  emi_1391/1 -> emi_1390/1
  cyemi_248/1 -> cfblk13/1(emi_2047)
  cfblk13/1(emi_2048) -> cyemi_254/1
  emi_2051/1 -> cfblk13/Action
  emi_2051/2 -> emi_2049/Action
  emi_2052/1 -> emi_2051/1

== system sampleModel7293_pp_1_1/cfblk171/cfblk11 ==
  cfblk1 : Inport
  cfblk6 : Inport  Port=2
  cfblk7 : Inport  Port=3
  Action Port : ActionPort  ActionType=else
  cfblk3 : simulink/Discrete/Transfer Fcn Real Zero  ZeroZ=0.75  ICPrevInput=0.0  DoSatur=off
      settings: SourceProductName=Simulink  SourceProductBaseCode=SL
  cfblk4 : DiscreteTransferFcn
  cfblk5 : DiscreteFilter
  cyemi_265 : DataTypeConversion  OutDataTypeStr=double
  cyemi_266 : DataTypeConversion  OutDataTypeStr=double
  cyemi_267 : DataTypeConversion  OutDataTypeStr=double
  cfblk2 : Outport
  cfblk8 : Outport  Port=2
  wires:
  cfblk4/1 -> cfblk2/1
  cfblk5/1 -> cfblk8/1
  cyemi_265/1 -> cfblk3/1
  cfblk7/1 -> cyemi_265/1
  cyemi_266/1 -> cfblk4/1
  cfblk1/1 -> cyemi_266/1
  cyemi_267/1 -> cfblk5/1
  cfblk6/1 -> cyemi_267/1

== system sampleModel7293_pp_1_1/cfblk171/cfblk15 ==
  emi_1941 : Inport
  Action Port : ActionPort  ActionType=then
  cfblk15 : Delay
  emi_1942 : Outport
  wires:
  emi_1941/1 -> cfblk15/1
  cfblk15/1 -> emi_1942/1

== system sampleModel7293_pp_1_1/cfblk171/cfblk4 ==
  emi_674 : Inport
  Action Port : ActionPort  ActionType=then
  cfblk4 : DiscreteStateSpace  SampleTime=-1
  emi_675 : Outport
  wires:
  emi_674/1 -> cfblk4/1
  cfblk4/1 -> emi_675/1

== system sampleModel7293_pp_1_1/cfblk171/cfblk5 ==
  emi_171 : Inport
  Action Port : ActionPort  ActionType=then
  cfblk5 : DiscreteStateSpace  SampleTime=-1
  emi_172 : Outport
  wires:
  emi_171/1 -> cfblk5/1
  cfblk5/1 -> emi_172/1

== system sampleModel7293_pp_1_1/cfblk171/emi_173 ==
  Action Port : ActionPort  ActionType=else
  emi_174 : Assertion

== system sampleModel7293_pp_1_1/cfblk171/emi_1943 ==
  Action Port : ActionPort  ActionType=else
  emi_1944 : Assertion

== system sampleModel7293_pp_1_1/cfblk171/emi_676 ==
  Action Port : ActionPort  ActionType=else
  emi_677 : Assertion

== system sampleModel7293_pp_1_1/cfblk172/cfblk7 ==
  emi_973 : Inport
  Action Port : ActionPort  ActionType=then
  cfblk7 : simulink/Continuous/PID Controller  Controller=PID  TimeDomain=Discrete-time  SampleTime=-1  IntegratorMethod=Forward Euler  FilterMethod=Forward Euler  Form=Parallel  UseFilter=on  ControllerParametersSource=internal  P=1  I=1  D=0  N=100  InitialConditionSource=internal  InitialConditionForIntegrator=0  InitialConditionForFilter=0  ExternalReset=none  LimitOutput=off  UpperSaturationLimit=inf  LowerSaturationLimit=-inf  LinearizeAsGain=off  AntiWindupMode=none  Kb=1  TrackingMode=off  Kt=1  PParamMin=[]  PParamMax=[]  IParamMin=[]  IParamMax=[]  DParamMin=[]  DParamMax=[]  NParamMin=[]  NParamMax=[]  KbParamMin=[]  KbParamMax=[]  KtParamMin=[]  KtParamMax=[]  POutMin=[]  POutMax=[]  IOutMin=[]  IOutMax=[]  DOutMin=[]  DOutMax=[]  NOutMin=[]  NOutMax=[]  KbOutMin=[]  KbOutMax=[]  KtOutMin=[]  KtOutMax=[]  IntegratorOutMin=[]  IntegratorOutMax=[]  FilterOutMin=[]  FilterOutMax=[]  SumOutMin=[]  SumOutMax=[]  SumI1OutMin=[]  SumI1OutMax=[]  SumI2OutMin=[]  SumI2OutMax=[]  SumI3OutMin=[]  SumI3OutMax=[]  SumDOutMin=[]  SumDOutMax=[]  SaturationOutMin=[]  SaturationOutMax=[]  IntegratorContinuousStateAttributes=''  IntegratorStateMustResolveToSignalObject=off  IntegratorRTWStateStorageClass=Auto  FilterContinuousStateAttributes=''  FilterStateMustResolveToSignalObject=off  FilterRTWStateStorageClass=Auto  DifferentiatorICPrevScaledInput=0  DifferentiatorOutMin=[]  DifferentiatorOutMax=[]  FilterDiffOutCoefMin=[]  FilterDiffOutCoefMax=[]  SumDenOutMin=[]  SumDenOutMax=[]  SumNumOutMin=[]  SumNumOutMax=[]  ReciprocalOutMin=[]  ReciprocalOutMax=[]  DivideOutMin=[]  DivideOutMax=[]  TunerSelectOption=Transfer Function Based (PID Tuner App)
  emi_974 : Outport
  wires:
  emi_973/1 -> cfblk7/1
  cfblk7/1 -> emi_974/1

== system sampleModel7293_pp_1_1/cfblk172/emi_975 ==
  Action Port : ActionPort  ActionType=else
  emi_976 : Assertion

== system sampleModel7293_pp_1_1/cfblk173/cfblk13 ==
  cfblk1 : Inport
  cfblk12 : Inport  Port=2
  Action Port : ActionPort  ActionType=then
  cfblk10 : Subsystem  TreatAsAtomicUnit=on
  cfblk11 : simulink/Discrete/Tapped Delay  vinit=0.0  samptime=-1  NumDelays=1  DelayOrder=Oldest  includeCurrent=off
  cfblk3 : DiscreteZeroPole  Poles=[0 0.5]  Gain=1  SampleTime=-1
  cfblk4 : Delay  DelayLengthSource=Input port
      settings: InputPortMap=u0,p1
  cfblk5 : DiscreteFir
  cfblk6 : DiscreteFir
  cfblk7 : simulink/Continuous/PID Controller  Controller=PID  TimeDomain=Discrete-time  SampleTime=-1  IntegratorMethod=Forward Euler  FilterMethod=Forward Euler  Form=Parallel  UseFilter=on  ControllerParametersSource=internal  P=1  I=1  D=0  N=100  InitialConditionSource=internal  InitialConditionForIntegrator=0  InitialConditionForFilter=0  ExternalReset=none  LimitOutput=off  UpperSaturationLimit=inf  LowerSaturationLimit=-inf  LinearizeAsGain=off  AntiWindupMode=none  Kb=1  TrackingMode=off  Kt=1  PParamMin=[]  PParamMax=[]  IParamMin=[]  IParamMax=[]  DParamMin=[]  DParamMax=[]  NParamMin=[]  NParamMax=[]  KbParamMin=[]  KbParamMax=[]  KtParamMin=[]  KtParamMax=[]  POutMin=[]  POutMax=[]  IOutMin=[]  IOutMax=[]  DOutMin=[]  DOutMax=[]  NOutMin=[]  NOutMax=[]  KbOutMin=[]  KbOutMax=[]  KtOutMin=[]  KtOutMax=[]  IntegratorOutMin=[]  IntegratorOutMax=[]  FilterOutMin=[]  FilterOutMax=[]  SumOutMin=[]  SumOutMax=[]  SumI1OutMin=[]  SumI1OutMax=[]  SumI2OutMin=[]  SumI2OutMax=[]  SumI3OutMin=[]  SumI3OutMax=[]  SumDOutMin=[]  SumDOutMax=[]  SaturationOutMin=[]  SaturationOutMax=[]  IntegratorContinuousStateAttributes=''  IntegratorStateMustResolveToSignalObject=off  IntegratorRTWStateStorageClass=Auto  FilterContinuousStateAttributes=''  FilterStateMustResolveToSignalObject=off  FilterRTWStateStorageClass=Auto  DifferentiatorICPrevScaledInput=0  DifferentiatorOutMin=[]  DifferentiatorOutMax=[]  FilterDiffOutCoefMin=[]  FilterDiffOutCoefMax=[]  SumDenOutMin=[]  SumDenOutMax=[]  SumNumOutMin=[]  SumNumOutMax=[]  ReciprocalOutMin=[]  ReciprocalOutMax=[]  DivideOutMin=[]  DivideOutMax=[]  TunerSelectOption=Transfer Function Based (PID Tuner App)
  cfblk8 : DiscreteTransferFcn
  cfblk9 : Subsystem  TreatAsAtomicUnit=on
  cyemi_{293..302} (10 alike) : DataTypeConversion  OutDataTypeStr=double
  emi_1073 : Subsystem  TreatAsAtomicUnit=on
  emi_1075 : If  IfExpression=Inf <= u1
  emi_1076 : DataTypeConversion  OutDataTypeStr=double
  emi_1716 : Subsystem  TreatAsAtomicUnit=on
  emi_1718 : If  IfExpression=Inf <= u1
  emi_1719 : DataTypeConversion  OutDataTypeStr=double
  cfblk2 : Outport
  wires:
  cfblk4/1 -> cfblk2/1
  cfblk6/1 -> cyemi_293/1, emi_1719/1
  cyemi_294/1 -> cfblk11/1
  cyemi_295/1 -> cfblk3/1
  cfblk5/1 -> cyemi_295/1
  cyemi_296/1 -> cfblk4/1
  cfblk12/1 -> cyemi_296/1
  cyemi_297/1 -> cfblk4/2
  cfblk8/1 -> cyemi_297/1, emi_1076/1
  cyemi_298/1 -> cfblk5/1
  cfblk11/1 -> cyemi_298/1
  cyemi_299/1 -> cfblk6/1
  cfblk7/1 -> cyemi_299/1
  cyemi_300/1 -> cfblk7/1
  cfblk1/1 -> cyemi_300/1
  cyemi_301/1 -> cfblk8/1
  cfblk3/1 -> cyemi_302/1
  cyemi_302/1 -> cfblk9/1(emi_1071)
  cfblk9/1(emi_1072) -> cyemi_301/1
  emi_1075/1 -> cfblk9/Action
  emi_1075/2 -> emi_1073/Action
  emi_1076/1 -> emi_1075/1
  cyemi_293/1 -> cfblk10/1(emi_1714)
  cfblk10/1(emi_1715) -> cyemi_294/1
  emi_1718/1 -> cfblk10/Action
  emi_1718/2 -> emi_1716/Action
  emi_1719/1 -> emi_1718/1

== system sampleModel7293_pp_1_1/cfblk173/cfblk14 ==
  cfblk1 : Inport
  cfblk7 : Inport  Port=2
  cfblk8 : Inport  Port=3
  Action Port : ActionPort  ActionType=else
  cfblk3 : Subsystem  TreatAsAtomicUnit=on
  cfblk4 : Subsystem  TreatAsAtomicUnit=on
  cfblk5 : DiscreteZeroPole  Poles=[0 0.5]  Gain=1  SampleTime=-1
  cfblk6 : DiscreteTransferFcn
  cfblk9 : Delay
  cyemi_{306..311} (6 alike) : DataTypeConversion  OutDataTypeStr=double
  emi_1986 : Subsystem  TreatAsAtomicUnit=on
  emi_1988 : If  IfExpression=0 <= u1
  emi_1989 : DataTypeConversion  OutDataTypeStr=double
  emi_841 : Subsystem  TreatAsAtomicUnit=on
  emi_843 : If  IfExpression=0 <= u1
  emi_844 : DataTypeConversion  OutDataTypeStr=double
  cfblk2 : Outport
  wires:
  cfblk5/1 -> cfblk2/1
  cfblk9/1 -> cyemi_307/1
  cfblk1/1 -> cyemi_308/1
  cyemi_309/1 -> cfblk5/1
  cfblk6/1 -> cyemi_309/1, emi_844/1
  cyemi_310/1 -> cfblk6/1
  cfblk8/1 -> cyemi_310/1
  cyemi_311/1 -> cfblk9/1
  cyemi_306/1 -> cfblk3/1(emi_839)
  cfblk3/1(emi_840) -> cyemi_311/1, emi_1989/1
  emi_843/1 -> cfblk3/Action
  emi_843/2 -> emi_841/Action
  emi_844/1 -> emi_843/1
  cyemi_307/1 -> cfblk4/1(emi_1983)
  cyemi_308/1 -> cfblk4/2(emi_1984)
  cfblk4/1(emi_1985) -> cyemi_306/1
  emi_1988/1 -> cfblk4/Action
  emi_1988/2 -> emi_1986/Action
  emi_1989/1 -> emi_1988/1

== system sampleModel7293_pp_1_1/cfblk174/cfblk3 ==
  emi_617 : Inport
  Action Port : ActionPort  ActionType=then
  cfblk3 : simulink/Continuous/PID Controller  Controller=PID  TimeDomain=Discrete-time  SampleTime=-1  IntegratorMethod=Forward Euler  FilterMethod=Forward Euler  Form=Parallel  UseFilter=on  ControllerParametersSource=internal  P=1  I=1  D=0  N=100  InitialConditionSource=internal  InitialConditionForIntegrator=0  InitialConditionForFilter=0  ExternalReset=none  LimitOutput=off  UpperSaturationLimit=inf  LowerSaturationLimit=-inf  LinearizeAsGain=off  AntiWindupMode=none  Kb=1  TrackingMode=off  Kt=1  PParamMin=[]  PParamMax=[]  IParamMin=[]  IParamMax=[]  DParamMin=[]  DParamMax=[]  NParamMin=[]  NParamMax=[]  KbParamMin=[]  KbParamMax=[]  KtParamMin=[]  KtParamMax=[]  POutMin=[]  POutMax=[]  IOutMin=[]  IOutMax=[]  DOutMin=[]  DOutMax=[]  NOutMin=[]  NOutMax=[]  KbOutMin=[]  KbOutMax=[]  KtOutMin=[]  KtOutMax=[]  IntegratorOutMin=[]  IntegratorOutMax=[]  FilterOutMin=[]  FilterOutMax=[]  SumOutMin=[]  SumOutMax=[]  SumI1OutMin=[]  SumI1OutMax=[]  SumI2OutMin=[]  SumI2OutMax=[]  SumI3OutMin=[]  SumI3OutMax=[]  SumDOutMin=[]  SumDOutMax=[]  SaturationOutMin=[]  SaturationOutMax=[]  IntegratorContinuousStateAttributes=''  IntegratorStateMustResolveToSignalObject=off  IntegratorRTWStateStorageClass=Auto  FilterContinuousStateAttributes=''  FilterStateMustResolveToSignalObject=off  FilterRTWStateStorageClass=Auto  DifferentiatorICPrevScaledInput=0  DifferentiatorOutMin=[]  DifferentiatorOutMax=[]  FilterDiffOutCoefMin=[]  FilterDiffOutCoefMax=[]  SumDenOutMin=[]  SumDenOutMax=[]  SumNumOutMin=[]  SumNumOutMax=[]  ReciprocalOutMin=[]  ReciprocalOutMax=[]  DivideOutMin=[]  DivideOutMax=[]  TunerSelectOption=Transfer Function Based (PID Tuner App)
  emi_618 : Outport
  wires:
  emi_617/1 -> cfblk3/1
  cfblk3/1 -> emi_618/1

== system sampleModel7293_pp_1_1/cfblk174/cfblk6 ==
  emi_596 : Inport
  Action Port : ActionPort  ActionType=then
  cfblk6 : DiscreteZeroPole  Poles=[0 0.5]  Gain=1  SampleTime=-1
  emi_597 : Outport
  wires:
  emi_596/1 -> cfblk6/1
  cfblk6/1 -> emi_597/1

== system sampleModel7293_pp_1_1/cfblk174/emi_598 ==
  Action Port : ActionPort  ActionType=else
  emi_599 : Assertion

== system sampleModel7293_pp_1_1/cfblk174/emi_619 ==
  Action Port : ActionPort  ActionType=else
  emi_620 : Assertion

== system sampleModel7293_pp_1_1/cfblk175/cfblk16 ==
  cfblk1 : Inport
  Action Port : ActionPort  ActionType=then
  cfblk10 : Delay
  cfblk3 : Subsystem  TreatAsAtomicUnit=on
  cfblk4 : Delay  DelayLengthSource=Input port
      settings: InputPortMap=u0,p1
  cfblk5 : simulink/Discrete/Transfer Fcn First Order  PoleZ=0.95  ICPrevOutput=0.0  DoSatur=off
      settings: SourceProductName=Simulink
  cfblk6 : Subsystem  TreatAsAtomicUnit=on
  cfblk7 : UnitDelay  SampleTime=-1
  cfblk8 : DiscreteTransferFcn
  cfblk9 : simulink/Discrete/Transfer Fcn Lead or Lag  PoleZ=0.95  ZeroZ=0.75  ICPrevOutput=0.0  ICPrevInput=0.0  DoSatur=off
      settings: SourceProductName=Simulink  SourceProductBaseCode=SL
  cyemi_{333..334,336..337} (4 alike) : DataTypeConversion  OutDataTypeStr=uint32
  cyemi_{335,338..341} (5 alike) : DataTypeConversion  OutDataTypeStr=double
  emi_1087 : Subsystem  TreatAsAtomicUnit=on
  emi_1089 : If  IfExpression=Inf <= u1
  emi_1090 : DataTypeConversion  OutDataTypeStr=double
  emi_1254 : Subsystem  TreatAsAtomicUnit=on
  emi_1256 : If  IfExpression=Inf <= u1
  emi_1257 : DataTypeConversion  OutDataTypeStr=double
  cfblk2 : Outport
  wires:
  cfblk8/1 -> cfblk2/1, emi_1257/1
  cyemi_333/1 -> cfblk10/1
  cfblk5/1 -> cyemi_333/1
  cfblk10/1 -> cyemi_334/1
  cyemi_335/1 -> cfblk4/1
  cfblk7/1 -> cyemi_335/1, emi_1090/1
  cyemi_336/1 -> cfblk4/2
  cyemi_337/1 -> cfblk5/1
  cfblk9/1 -> cyemi_338/1
  cyemi_339/1 -> cfblk7/1
  cfblk1/1 -> cyemi_339/1
  cyemi_340/1 -> cfblk8/1
  cyemi_341/1 -> cfblk9/1
  cfblk4/1 -> cyemi_341/1
  cyemi_334/1 -> cfblk3/1(emi_1085)
  cfblk3/1(emi_1086) -> cyemi_337/1, cyemi_336/1
  emi_1089/1 -> cfblk3/Action
  emi_1089/2 -> emi_1087/Action
  emi_1090/1 -> emi_1089/1
  cyemi_338/1 -> cfblk6/1(emi_1252)
  cfblk6/1(emi_1253) -> cyemi_340/1
  emi_1256/1 -> cfblk6/Action
  emi_1256/2 -> emi_1254/Action
  emi_1257/1 -> emi_1256/1
